simulink model "LIM_model_controller"  (R2021a)
settings: Solver=FixedStepAuto  StartTime=0.0  StopTime=8.5  FixedStep=1e-4  RelTol=1e-6
values from neighbouring files (symbols this model uses):
  l = 0.308    [LIMvariables.m]
  Lm = 0.0416    [LIM_parameters.m]    (also in LIMvariables.m = 0.0376)
  Lx = Lm+Llx    (= 0.0601)    [LIMvariables.m]
  Ly = Lm+Lly    (= 0.0441)    [LIMvariables.m]
  m = 10    [LIM_parameters.m]    (also in LIMvariables.m)
  P = 4400    [LIMvariables.m]
  Rx = 1.2    [LIMvariables.m]
  Ry = 2.7    [LIMvariables.m]
  tau = L/p    (= 0.25)    [LIM_parameters.m]    (also in LIMvariables.m = 0.066)
  Ty = Ly/Ry    (= 0.0163333333333)    [LIMvariables.m]
  we = 314.16    [LIMvariables.m]
libraries: slpidlib x5, simulink x3
settings Model: Creator=Asus  LastModifiedBy=Asus

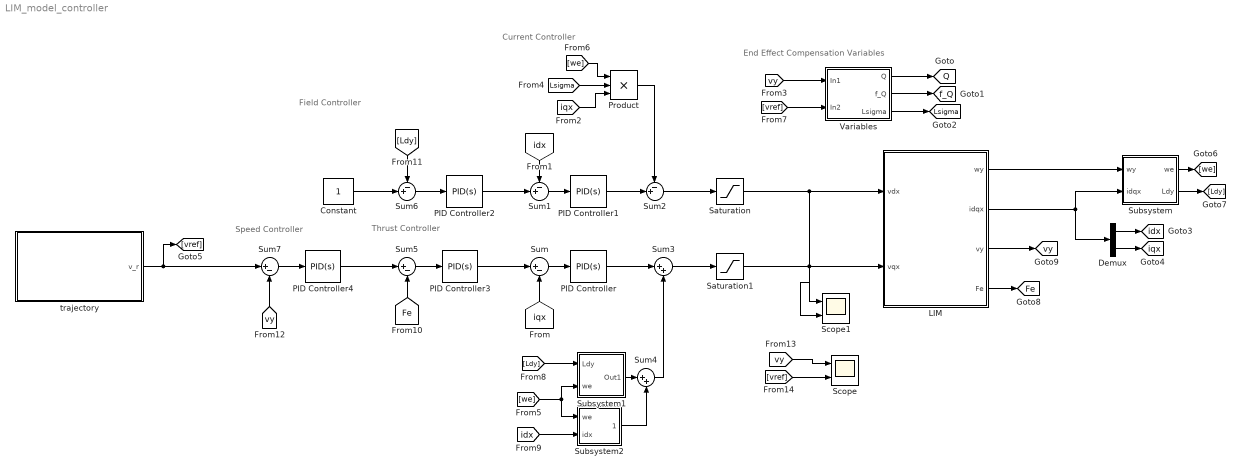
== system LIM_model_controller ==
  note: End Effect Compensation Variables
  note: Field Controller
  note: Speed Controller
  note: Thrust Controller
  note: Current Controller
  Constant : Constant
  Demux : Demux  Outputs=2
  LIM : Subsystem
  PID Controller{,1..4} (5 alike) : slpidlib/PID Controller  Controller=PID  Form=Parallel  TimeDomain=Continuous-time  UseExternalTs=off  SampleTime=-1  IntegratorMethod=Forward Euler  FilterMethod=Forward Euler  ControllerParametersSource=internal  P=1  I=1  D=0  UseFilter=on  N=100  TunerSelectOption=Transfer Function Based (PID Tuner App)  InitialConditionSource=internal  InitialConditionForIntegrator=0  InitialConditionForFilter=0  DifferentiatorICPrevScaledInput=0  ExternalReset=none  TrackingMode=off  Kt=1  LimitOutput=off  SatLimitsSource=internal  UpperSaturationLimit=inf  LowerSaturationLimit=-inf  LinearizeAsGain=on  AntiWindupMode=none  Kb=1  POutMin=[]  POutMax=[]  IOutMin=[]  IOutMax=[]  DOutMin=[]  DOutMax=[]  NOutMin=[]  NOutMax=[]  SumOutMin=[]  SumOutMax=[]  SaturationOutMin=[]  SaturationOutMax=[]  PParamMin=[]  PParamMax=[]  IParamMin=[]  IParamMax=[]  DParamMin=[]  DParamMax=[]  NParamMin=[]  NParamMax=[]  KbParamMin=[]  KbParamMax=[]  KtParamMin=[]  KtParamMax=[]  KbOutMin=[]  KbOutMax=[]  KtOutMin=[]  KtOutMax=[]  IntegratorOutMin=[]  IntegratorOutMax=[]  FilterOutMin=[]  FilterOutMax=[]  SumI1OutMin=[]  SumI1OutMax=[]  SumI2OutMin=[]  SumI2OutMax=[]  SumI3OutMin=[]  SumI3OutMax=[]  SumI4OutMin=[]  SumI4OutMax=[]  SumDOutMin=[]  SumDOutMax=[]  DifferentiatorOutMin=[]  DifferentiatorOutMax=[]  FilterDiffOutCoefMin=[]  FilterDiffOutCoefMax=[]  ReciprocalOutMin=[]  ReciprocalOutMax=[]  SumDenOutMin=[]  SumDenOutMax=[]  SumNumOutMin=[]  SumNumOutMax=[]  DivideOutMin=[]  DivideOutMax=[]  UdiffTsProdOutMin=[]  UdiffTsProdOutMax=[]  NTsProdOutMin=[]  NTsProdOutMax=[]  UintegralTsProdOutMin=[]  UintegralTsProdOutMax=[]  UngainTsProdOutMin=[]  UngainTsProdOutMax=[]  IntegratorContinuousStateAttributes=''  IntegratorStateMustResolveToSignalObject=off  IntegratorRTWStateStorageClass=Auto  FilterContinuousStateAttributes=''  FilterStateMustResolveToSignalObject=off  FilterRTWStateStorageClass=Auto  ParallelPVariant=InternalParameters  IdealPVariant=Disabled  IVariant=InternalParameters  DVariant=InternalParameters  IntegratorVariant=Continuous  SatVariant=Disabled  AWVariant=Passthrough  PCopyVariant=Disabled  TRVariant=Disabled  FdbkBlocksVariant=Forward  IdealPFdbkVariant=Disabled  SatFdbkVariant=Disabled  DerivativeFilterVariant=ContFilter  NVariant=InternalParameters  NCopyVariant=Disabled  FilterICVariant=InternalICsFilter  IntegratorICVariant=InternalICs  ExternalResetVariant=Disabled  TRSumVariant=Passthrough  SumFdbkVariant=Disabled  SumVariant=Sum_PID  TsampFilterVariant=InternalTs  TsampNgainVariant=Passthrough  TsampIntegralVariant=Passthrough  ExternalSaturationOutDataTypeStr=Inherit: Same as second input
  Product : Product  Inputs=3
  Saturation : Saturate  UpperLimit=100  LowerLimit=-100
  Saturation1 : Saturate  UpperLimit=100  LowerLimit=-100
  Scope : Scope  NumInputPorts=2
  Scope1 : Scope  NumInputPorts=2
  Subsystem : Subsystem
  Subsystem1 : Subsystem
  Subsystem2 : Subsystem
  Sum : Sum  Inputs=|+-
  Sum1 : Sum  Inputs=-+|
  Sum2 : Sum  Inputs=-+|
  Sum3 : Sum  Inputs=|++
  Sum4 : Sum  Inputs=|++
  Sum5 : Sum  Inputs=|+-
  Sum6 : Sum  Inputs=-+|
  Sum7 : Sum  Inputs=|+-
  Variables : Subsystem
  trajectory : Subsystem
  tag scope: Fe=global, Lsigma=global, Q=global, f_Q=global, idx=global, iqx=global, vy=global
  wires:
  [vref] -> Variables/2(In2)
  Variables/2(f_Q) -> [f_Q]
  Variables/3(Lsigma) -> [Lsigma]
  Variables/1(Q) -> [Q]
  [vy] -> Variables/1(In1)
  trajectory/1(v_r) -> Sum7/1, [vref]
  LIM/3(vy) -> [vy]
  Sum/1 -> PID Controller/1
  Sum1/1 -> PID Controller1/1
  Saturation1/1 -> Scope1/2, LIM/2(vqx)
  Saturation/1 -> Scope1/1, LIM/1(vdx)
  [iqx] -> Sum/2
  [idx] -> Sum1/1
  Sum2/1 -> Saturation/1
  PID Controller1/1 -> Sum2/2
  LIM/1(wy) -> Subsystem/1(wy)
  LIM/2(idqx) -> Subsystem/2(idqx), Demux/1
  Demux/1 -> [idx]
  Demux/2 -> [iqx]
  Subsystem/1(we) -> [we]
  [we] -> Product/1
  [Lsigma] -> Product/2
  [iqx] -> Product/3
  Product/1 -> Sum2/1
  Subsystem/2(Ldy) -> [Ldy]
  Sum3/1 -> Saturation1/1
  PID Controller/1 -> Sum3/1
  Subsystem2/1(Out1) -> Sum4/2
  Subsystem1/1(Out1) -> Sum4/1
  Sum4/1 -> Sum3/2
  [Ldy] -> Subsystem1/1(Ldy)
  [idx] -> Subsystem2/2(idx)
  [we] -> Subsystem1/2(we), Subsystem2/1(we)
  LIM/4(Fe) -> [Fe]
  PID Controller3/1 -> Sum/1
  PID Controller2/1 -> Sum1/2
  Sum5/1 -> PID Controller3/1
  Sum6/1 -> PID Controller2/1
  [Fe] -> Sum5/2
  [Ldy] -> Sum6/1
  Constant/1 -> Sum6/2
  PID Controller4/1 -> Sum5/1
  [vy] -> Sum7/2
  Sum7/1 -> PID Controller4/1
  [vy] -> Scope/1
  [vref] -> Scope/2

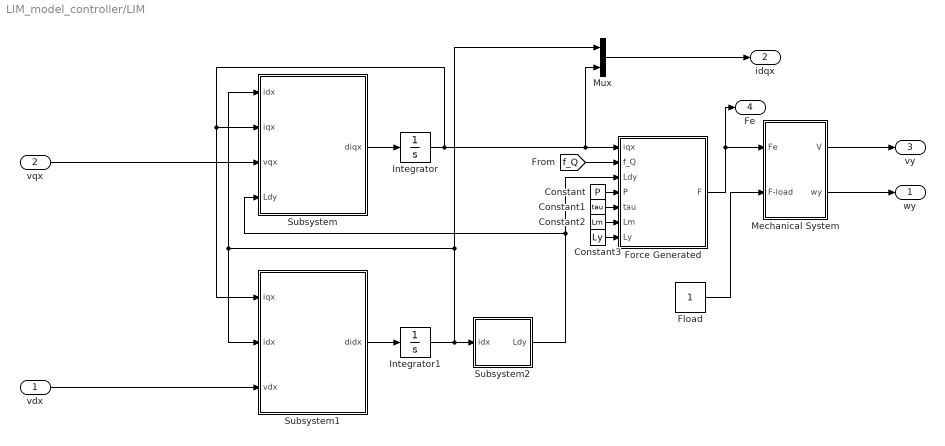
== system LIM_model_controller/LIM ==
  vdx : Inport
  vqx : Inport  Port=2
  Constant : Constant  Value=P
  Constant1 : Constant  Value=tau
  Constant2 : Constant  Value=Lm
  Constant3 : Constant  Value=Ly
  Fload : Constant
  Force Generated : MATLAB Function  TreatAsAtomicUnit=on
  Integrator : Integrator  InitialCondition=0.1
  Integrator1 : Integrator
  Mechanical System : Subsystem
  Mux : Mux  Inputs=2
  Subsystem : Subsystem
  Subsystem1 : Subsystem
  Subsystem2 : Subsystem
  wy : Outport
  idqx : Outport  Port=2
  vy : Outport  Port=3
  Fe : Outport  Port=4
  wires:
  Integrator/1 -> Subsystem1/1(iqx), Subsystem/2(iqx), Mux/2, Force Generated/1(iqx)
  Subsystem/1(diqx) -> Integrator/1
  vdx/1 -> Subsystem1/3(vdx)
  Integrator1/1 -> Subsystem2/1(idx), Mux/1, Subsystem1/2(idx), Subsystem/1(idx)
  Fload/1 -> Mechanical System/2(F-load)
  Subsystem1/1(didx) -> Integrator1/1
  Subsystem2/1(Ldy) -> Subsystem/4(Ldy), Force Generated/3(Ldy)
  Force Generated/1(F) -> Mechanical System/1(Fe), Fe/1
  [f_Q] -> Force Generated/2(f_Q)
  Mechanical System/2(wy) -> wy/1
  Mechanical System/1(V) -> vy/1
  vqx/1 -> Subsystem/3(vqx)
  Mux/1 -> idqx/1
  Constant/1 -> Force Generated/4(P)
  Constant1/1 -> Force Generated/5(tau)
  Constant2/1 -> Force Generated/6(Lm)
  Constant3/1 -> Force Generated/7(Ly)

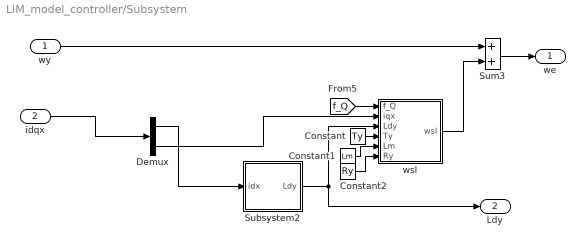
== system LIM_model_controller/Subsystem ==
  wy : Inport
  idqx : Inport  Port=2
  Constant : Constant  Value=Ty
  Constant1 : Constant  Value=Lm
  Constant2 : Constant  Value=Ry
  Demux : Demux  Outputs=2
  Subsystem2 : Subsystem
  Sum3 : Sum
  wsl : MATLAB Function  TreatAsAtomicUnit=on
  we : Outport
  Ldy : Outport  Port=2
  wires:
  Subsystem2/1(Ldy) -> Ldy/1, wsl/3(Ldy)
  Demux/2 -> wsl/2(iqx)
  Demux/1 -> Subsystem2/1(idx)
  [f_Q] -> wsl/1(f_Q)
  idqx/1 -> Demux/1
  wsl/1(wsl) -> Sum3/2
  Sum3/1 -> we/1
  wy/1 -> Sum3/1
  Constant/1 -> wsl/4(Ty)
  Constant1/1 -> wsl/5(Lm)
  Constant2/1 -> wsl/6(Ry)

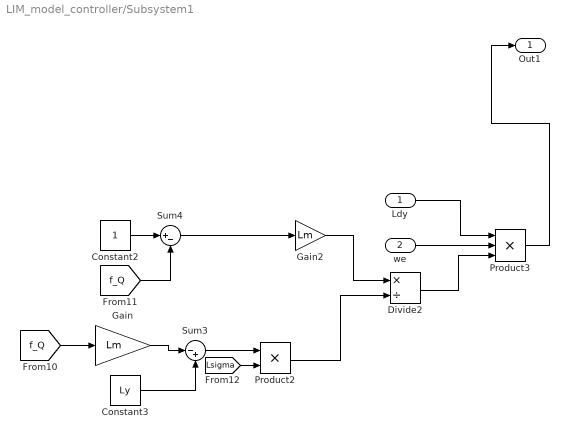
== system LIM_model_controller/Subsystem1 ==
  Ldy : Inport
  we : Inport  Port=2
  Constant2 : Constant
  Constant3 : Constant  Value=Ly
  Divide2 : Product  Inputs=*/
  Gain : Gain  Gain=Lm
  Gain2 : Gain  Gain=Lm
  Product2 : Product
  Product3 : Product  Inputs=3
  Sum3 : Sum  Inputs=|-+
  Sum4 : Sum  Inputs=|+-
  Out1 : Outport
  wires:
  [f_Q] -> Gain/1
  Constant3/1 -> Sum3/2
  Sum3/1 -> Product2/1
  Sum4/1 -> Gain2/1
  [Lsigma] -> Product2/2
  Constant2/1 -> Sum4/1
  Ldy/1 -> Product3/1
  [f_Q] -> Sum4/2
  Product2/1 -> Divide2/2
  Divide2/1 -> Product3/3
  Gain2/1 -> Divide2/1
  Gain/1 -> Sum3/1
  we/1 -> Product3/2
  Product3/1 -> Out1/1

== system LIM_model_controller/Subsystem2 ==
  we : Inport
  idx : Inport  Port=2
  Product1 : Product  Inputs=3
  Out1 : Outport
  wires:
  idx/1 -> Product1/3
  [Lsigma] -> Product1/2
  Product1/1 -> Out1/1
  we/1 -> Product1/1

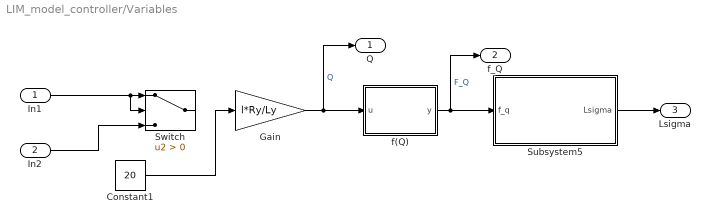
== system LIM_model_controller/Variables ==
  In1 : Inport
  In2 : Inport  Port=2
  Constant1 : Constant  Value=20
  Gain : Gain  Gain=l*Ry/Ly
  Subsystem5 : Subsystem
  Switch : Switch  Criteria=u2 > Threshold
  f(Q) : MATLAB Function  TreatAsAtomicUnit=on
  Q : Outport
  f_Q : Outport  Port=2
  Lsigma : Outport  Port=3
  wires:
  In1/1 -> Switch/2, Switch/1
  Gain/1 -> Q/1, f(Q)/1(u)  "Q"
  f(Q)/1(y) -> f_Q/1, Subsystem5/1(f_q)  "F_Q"
  Subsystem5/1(Lsigma) -> Lsigma/1
  In2/1 -> Switch/3
  Constant1/1 -> Gain/1

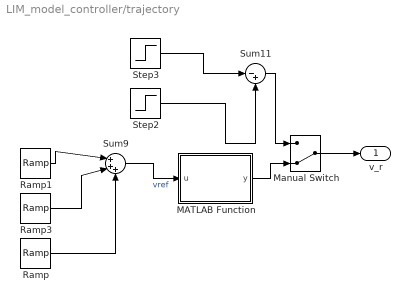
== system LIM_model_controller/trajectory ==
  MATLAB Function : MATLAB Function  TreatAsAtomicUnit=on
  Manual Switch : ManualSwitch  CurrentSetting=0
  Ramp : simulink/Sources/Ramp  slope=-6.5  start=5.28  InitialOutput=0
  Ramp1 : simulink/Sources/Ramp  slope=4.12  start=0  InitialOutput=0.1
  Ramp3 : simulink/Sources/Ramp  slope=-4.4  start=5.28  InitialOutput=0.1
  Step2 : Step  Time=0  Before=0.1  After=20  SampleTime=0
  Step3 : Step  Time=4  Before=20  After=0.1  SampleTime=0
  Sum11 : Sum  Inputs=|-+
  Sum9 : Sum  Inputs=|+++
  v_r : Outport
  wires:
  MATLAB Function/1(y) -> Manual Switch/2
  Sum11/1 -> Manual Switch/1
  Ramp3/1 -> Sum9/2
  Step2/1 -> Sum11/2
  Ramp/1 -> Sum9/3
  Step3/1 -> Sum11/1
  Ramp1/1 -> Sum9/1
  Manual Switch/1 -> v_r/1
  Sum9/1 -> MATLAB Function/1(u)  "vref"

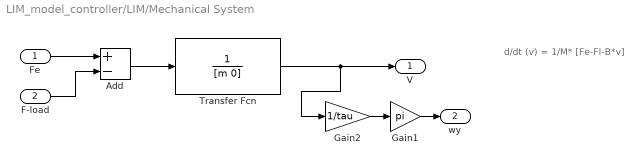
== system LIM_model_controller/LIM/Mechanical System ==
  note: d/dt (v) = 1/M* [Fe-Fl-B*v]
  Fe : Inport
  F-load : Inport  Port=2
  Add : Sum  Inputs=+-
  Gain1 : Gain  Gain=pi
  Gain2 : Gain  Gain=1/tau
  Transfer Fcn : TransferFcn  Denominator=[m 0]
  V : Outport
  wy : Outport  Port=2
  wires:
  Fe/1 -> Add/1
  F-load/1 -> Add/2
  Add/1 -> Transfer Fcn/1
  Gain2/1 -> Gain1/1
  Gain1/1 -> wy/1
  Transfer Fcn/1 -> Gain2/1, V/1

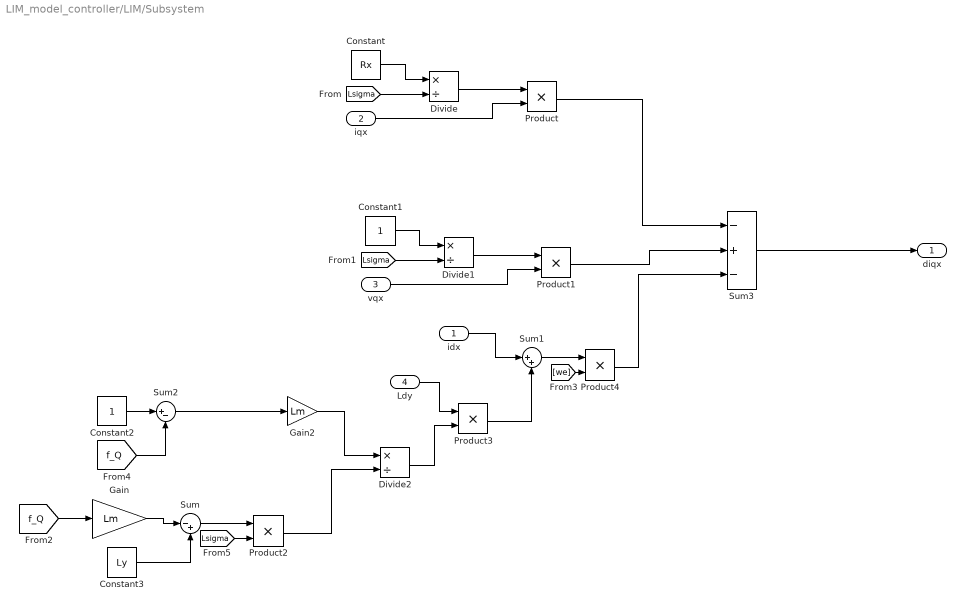
== system LIM_model_controller/LIM/Subsystem ==
  idx : Inport
  iqx : Inport  Port=2
  vqx : Inport  Port=3
  Ldy : Inport  Port=4
  Constant : Constant  Value=Rx
  Constant1 : Constant
  Constant2 : Constant
  Constant3 : Constant  Value=Ly
  Divide : Product  Inputs=*/
  Divide1 : Product  Inputs=*/
  Divide2 : Product  Inputs=*/
  Gain : Gain  Gain=Lm
  Gain2 : Gain  Gain=Lm
  Product{,1..4} (5 alike) : Product
  Sum : Sum  Inputs=|-+
  Sum1 : Sum  Inputs=|++
  Sum2 : Sum  Inputs=|+-
  Sum3 : Sum  Inputs=-+-
  diqx : Outport
  wires:
  Constant2/1 -> Sum2/1
  Gain/1 -> Sum/1
  Product3/1 -> Sum1/2
  Divide1/1 -> Product1/1
  Constant1/1 -> Divide1/1
  [Lsigma] -> Product2/2
  Ldy/1 -> Product3/1
  Sum/1 -> Product2/1
  Divide/1 -> Product/1
  Product1/1 -> Sum3/2
  Divide2/1 -> Product3/2
  Sum1/1 -> Product4/1
  Product/1 -> Sum3/1
  Product2/1 -> Divide2/2
  [Lsigma] -> Divide/2
  iqx/1 -> Product/2
  [f_Q] -> Sum2/2
  Gain2/1 -> Divide2/1
  Sum2/1 -> Gain2/1
  Sum3/1 -> diqx/1
  [f_Q] -> Gain/1
  Constant3/1 -> Sum/2
  vqx/1 -> Product1/2
  [Lsigma] -> Divide1/2
  Constant/1 -> Divide/1
  idx/1 -> Sum1/1
  Product4/1 -> Sum3/3
  [we] -> Product4/2

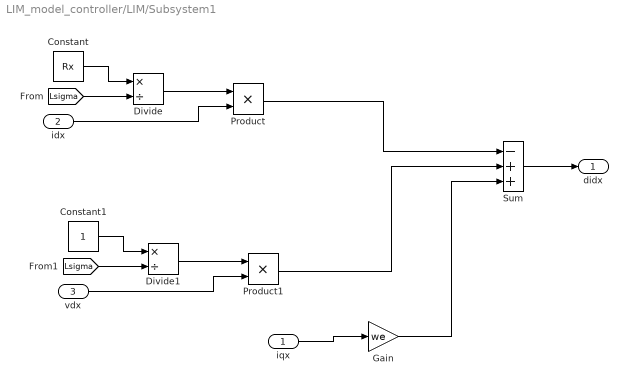
== system LIM_model_controller/LIM/Subsystem1 ==
  iqx : Inport
  idx : Inport  Port=2
  vdx : Inport  Port=3
  Constant : Constant  Value=Rx
  Constant1 : Constant
  Divide : Product  Inputs=*/
  Divide1 : Product  Inputs=*/
  Gain : Gain  Gain=we
  Product : Product
  Product1 : Product
  Sum : Sum  Inputs=-++
  didx : Outport
  wires:
  vdx/1 -> Product1/2
  Sum/1 -> didx/1
  [Lsigma] -> Divide1/2
  [Lsigma] -> Divide/2
  idx/1 -> Product/2
  Divide/1 -> Product/1
  Constant/1 -> Divide/1
  Gain/1 -> Sum/3
  Divide1/1 -> Product1/1
  Product/1 -> Sum/1
  Constant1/1 -> Divide1/1
  iqx/1 -> Gain/1
  Product1/1 -> Sum/2

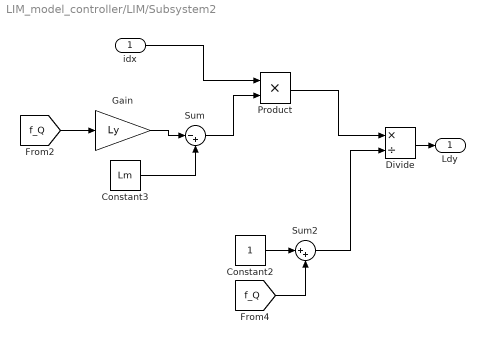
== system LIM_model_controller/LIM/Subsystem2 ==
  idx : Inport
  Constant2 : Constant
  Constant3 : Constant  Value=Lm
  Divide : Product  Inputs=*/
  Gain : Gain  Gain=Ly
  Product : Product
  Sum : Sum  Inputs=|-+
  Sum2 : Sum  Inputs=|++
  Ldy : Outport
  wires:
  Constant2/1 -> Sum2/1
  Product/1 -> Divide/1
  Gain/1 -> Sum/1
  Constant3/1 -> Sum/2
  idx/1 -> Product/1
  Divide/1 -> Ldy/1
  [f_Q] -> Sum2/2
  Sum/1 -> Product/2
  [f_Q] -> Gain/1
  Sum2/1 -> Divide/2

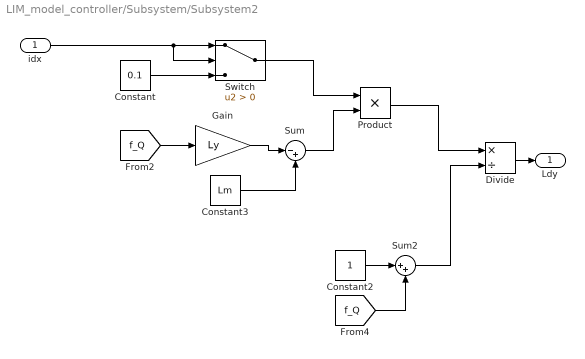
== system LIM_model_controller/Subsystem/Subsystem2 ==
  idx : Inport
  Constant : Constant  Value=0.1
  Constant2 : Constant
  Constant3 : Constant  Value=Lm
  Divide : Product  Inputs=*/
  Gain : Gain  Gain=Ly
  Product : Product
  Sum : Sum  Inputs=|-+
  Sum2 : Sum  Inputs=|++
  Switch : Switch  Criteria=u2 > Threshold
  Ldy : Outport
  wires:
  Constant2/1 -> Sum2/1
  Product/1 -> Divide/1
  Gain/1 -> Sum/1
  Constant3/1 -> Sum/2
  Divide/1 -> Ldy/1
  [f_Q] -> Sum2/2
  Sum/1 -> Product/2
  [f_Q] -> Gain/1
  Sum2/1 -> Divide/2
  idx/1 -> Switch/1, Switch/2
  Constant/1 -> Switch/3
  Switch/1 -> Product/1

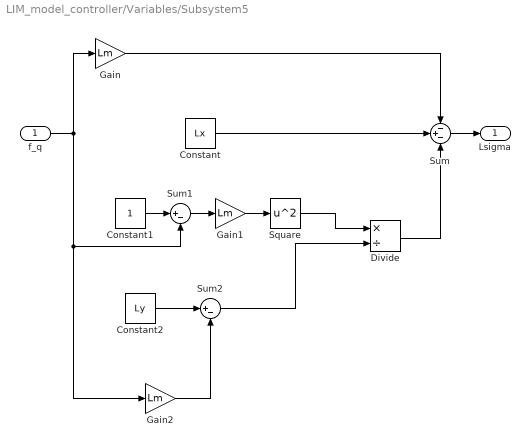
== system LIM_model_controller/Variables/Subsystem5 ==
  f_q : Inport
  Constant : Constant  Value=Lx
  Constant1 : Constant
  Constant2 : Constant  Value=Ly
  Divide : Product  Inputs=*/
  Gain : Gain  Gain=Lm
  Gain1 : Gain  Gain=Lm
  Gain2 : Gain  Gain=Lm
  Square : Math  Operator=square  SaturateOnIntegerOverflow=on
  Sum : Sum  Inputs=-+-
  Sum1 : Sum  Inputs=|+-
  Sum2 : Sum  Inputs=|+-
  Lsigma : Outport
  wires:
  Constant/1 -> Sum/2
  f_q/1 -> Sum1/2, Gain2/1, Gain/1
  Gain/1 -> Sum/1
  Sum/1 -> Lsigma/1
  Constant1/1 -> Sum1/1
  Sum1/1 -> Gain1/1
  Gain1/1 -> Square/1
  Square/1 -> Divide/1
  Constant2/1 -> Sum2/1
  Gain2/1 -> Sum2/2
  Sum2/1 -> Divide/2
  Divide/1 -> Sum/3

== matlab function LIM_model_controller/LIM/Force Generated ==
  data: iqx input; f_Q input; Ldy input; F output; P input; tau input; Lm input; Ly input
function F = fcn(iqx,f_Q,Ldy,P,tau,Lm,Ly)

F = ((3*P*pi)/2*2*tau)*(Lm*(1-f_Q)/(Ly-Lm*f_Q))*Ldy*iqx;

== matlab function LIM_model_controller/Variables/f(Q) ==
  data: u input; y output
function y = fcn(u)

y = (1-exp(-u))/u;

== matlab function LIM_model_controller/Subsystem/wsl ==
  data: f_Q input; wsl output; iqx input; Ldy input; Ty input; Lm input; Ry input
function wsl = fcn(f_Q,iqx,Ldy,Ty,Lm,Ry)

wsl = (Lm*(1-f_Q)*iqx)/((Ty-Lm*f_Q/Ry)*Ldy);

== matlab function LIM_model_controller/trajectory/MATLAB Function ==
  data: u input; y output
function y = fcn(u)

if u ~= 0
    y = u;
else
    y = 1;
end
